simulink model "simulation"  (R2016a)
settings: Solver=VariableStepAuto  StartTime=0.0  StopTime=100  RelTol=1e-3
values from neighbouring files (symbols this model uses):
  G = tf(wn^2,[1 2*zeta*wn wn^2 0])    [gen_bode.m]
  sin_freq = omega(i)    [gen_bode.m]
  Tdiscrete = 0.0001    [gen_bode.m]
  Tsim = 0.0001    [gen_bode.m]
settings Model: Creator=Black  LastModifiedBy=Black

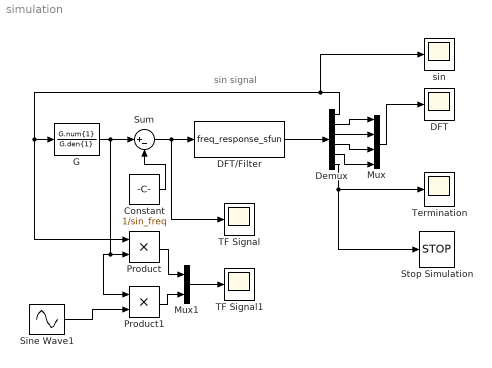
== system simulation ==
  note: sin signal
  Constant : Constant  Value=1/sin_freq
  DFT : Scope
  DFT/Filter : S-Function  FunctionName=freq_response_sfun  Parameters=Tdiscrete,Tsim,sin_freq  SFunctionDeploymentMode=off  EnableBusSupport=off
  Demux : Demux  Outputs=6
  G : TransferFcn  Numerator=G.num{1}  Denominator=G.den{1}
  Mux : Mux
  Mux1 : Mux  Inputs=2
  Product : Product
  Product1 : Product
  Sine Wave1 : Sin  Frequency=1000  Phase=pi/2  SampleTime=0
  Stop Simulation : Stop
  Sum : Sum  Inputs=|+-
  TF Signal : Scope
  TF Signal1 : Scope
  "Termination " : Scope
  sin : Scope
  wires:
  Demux/2 -> Mux/1
  Demux/3 -> Mux/2
  Demux/4 -> Mux/3
  Demux/5 -> Mux/4
  Demux/1 -> sin/1, G/1, Product/1
  DFT/Filter/1 -> Demux/1
  Mux/1 -> DFT/1
  Demux/6 -> Stop Simulation/1, "Termination "/1
  Sine Wave1/1 -> Product1/2
  Product1/1 -> Mux1/2
  Product/1 -> Mux1/1
  Mux1/1 -> TF Signal1/1
  Constant/1 -> Sum/2
  G/1 -> Product1/1, Product/2, Sum/1
  Sum/1 -> TF Signal/1, DFT/Filter/1
